simulink model "ME425HW2SIMULINK"  (R2024b)
settings: Solver=VariableStepAuto  StartTime=0.0  StopTime=simTime  RelTol=1e-3
values from neighbouring files (symbols this model uses):
  alpha_initial = pi/6    (= 0.523598775598)    [ME425HW2MATLAB.m]
  beta_initial = -pi/12    (= -0.261799387799)    [ME425HW2MATLAB.m]
  k_alpha = 3    [ME425HW2MATLAB.m]
  k_beta = -1    [ME425HW2MATLAB.m]
  k_rho = 0.45    [ME425HW2MATLAB.m]
  rho_initial = 0.5    [ME425HW2MATLAB.m]
settings Model: Creator=Arda Gencer  LastModifiedBy=Arda Gencer

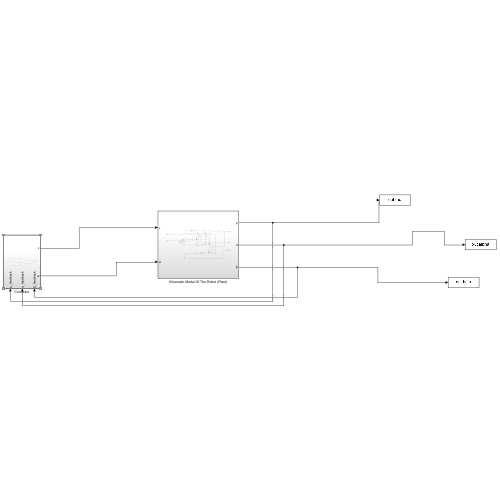
[thumbnail: Simulink's stored preview of the top-level diagram]
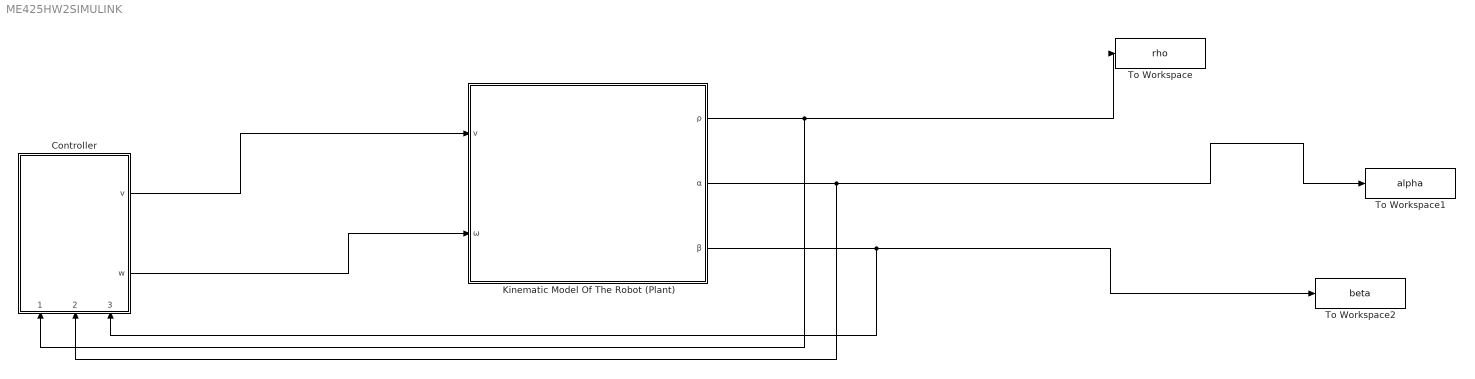
== system ME425HW2SIMULINK ==
  Controller : Subsystem
      settings: PortSchema="{\"entries\":[{\"content\":{\"sides\":[{\"content\":{},\"type\":\"ConnectorPlacement.EquallySpacedRectSide\",\"uuid\":\"75375935-2868-4b1b-a242-ab1ccb8ca21c\"},{\"content\":{\"connectorIds\":[\"Out1\",\"Out2\"],\"side\":\"RIGHT\"},\"type\":\"ConnectorPlacement.EquallySpacedRectSide\",\"uuid\":\"ed5a361e-a2c2-488a-aca6-bd0afa006ee2\"},{\"content\":{\"side\":\"TOP\"},\"type\":\"ConnectorPlacement.EquallySpacedRectSide\",\"uuid\":\"b9b83b9d-1c68-4626-97af-6a3bec3390e5\"},{\"content\":{\"connectorIds\":[\"In1\",\"In2\",\"In3\"],\"side\":\"BOTTOM\"},\"type\":\"ConnectorPlacement.EquallySpacedRectSide\",\"uuid\":\"91ac679b-6217-4ff3-855f-ef24c0e6137b\"}]},\"type\":\"ConnectorPlacement.EquallySpacedConnector\",\"uuid\":\"711fb22c-f1e8-402d-b054-03d08cfeb706\"}],\"packageUris\":[\"http://schema.mathworks.com/mf0/Connector/R2020b\"],\"version\":\"1.0\"}"
  Kinematic Model Of The Robot (Plant) : Subsystem
  To Workspace : ToWorkspace  VariableName=rho  SampleTime=-1
  To Workspace1 : ToWorkspace  VariableName=alpha  SampleTime=-1
  To Workspace2 : ToWorkspace  VariableName=beta  SampleTime=-1
  wires:
  Kinematic Model Of The Robot (Plant)/2(α) -> Controller/2(α_feedback), To Workspace1/1
  Kinematic Model Of The Robot (Plant)/1(ρ) -> Controller/1(ρ_feedback), To Workspace/1
  Kinematic Model Of The Robot (Plant)/3(β) -> Controller/3(β_feedback), To Workspace2/1
  Controller/1(v) -> Kinematic Model Of The Robot (Plant)/1(v)
  Controller/2(w) -> Kinematic Model Of The Robot (Plant)/2(ω)

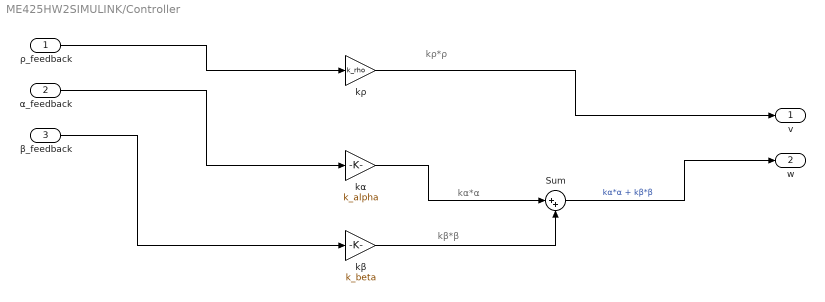
== system ME425HW2SIMULINK/Controller ==
  note: kβ*β
  note: kα*α
  note: kρ*ρ
  ρ_feedback : Inport
  α_feedback : Inport  Port=2
  β_feedback : Inport  Port=3
  Sum : Sum  Inputs=|++
  kα : Gain  Gain=k_alpha
  kβ : Gain  Gain=k_beta
  kρ : Gain  Gain=k_rho
  v : Outport
  w : Outport  Port=2
  wires:
  ρ_feedback/1 -> kρ/1
  kρ/1 -> v/1
  α_feedback/1 -> kα/1
  β_feedback/1 -> kβ/1
  kα/1 -> Sum/1
  kβ/1 -> Sum/2
  Sum/1 -> w/1  "kα*α + kβ*β"

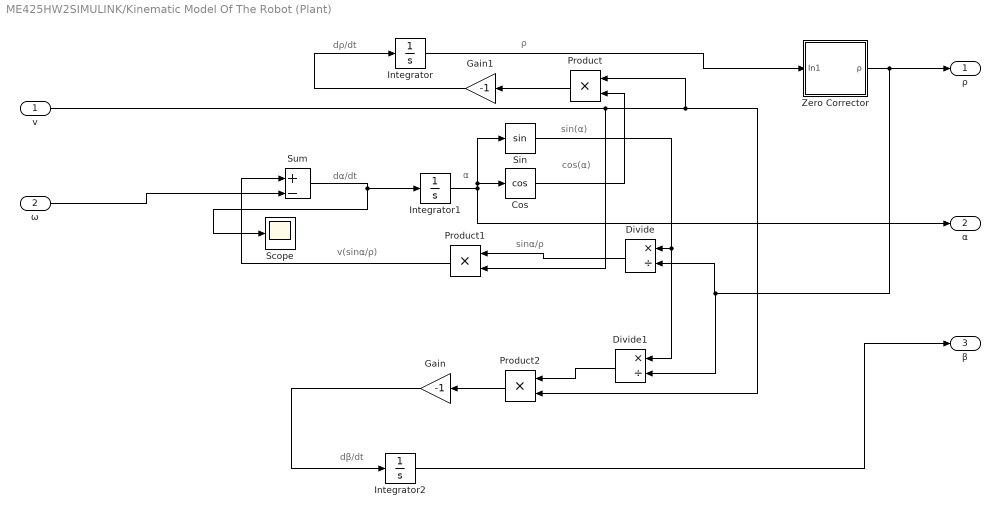
== system ME425HW2SIMULINK/Kinematic Model Of The Robot (Plant) ==
  note: dβ/dt
  note: sin(α)
  note: v(sinα/ρ)
  note: sinα/ρ
  note: ρ
  note: dα/dt
  note: dρ/dt
  note: cos(α)
  note: α
  v : Inport
  ω : Inport  Port=2
  Cos : Trigonometry  Operator=cos
  Divide : Product  Inputs=*/
  Divide1 : Product  Inputs=*/
  Gain : Gain  Gain=-1
  Gain1 : Gain  Gain=-1
  Integrator : Integrator  InitialCondition=rho_initial
  Integrator1 : Integrator  InitialCondition=alpha_initial  WrappedStateUpperValue=2*pi  WrappedStateLowerValue=0
  Integrator2 : Integrator  InitialCondition=beta_initial  WrappedStateUpperValue=2*pi  WrappedStateLowerValue=0
  Product : Product
  Product1 : Product
  Product2 : Product
  Scope : Scope
  Sin : Trigonometry
  Sum : Sum  Inputs=|+-
  Zero Corrector : Subsystem
  ρ : Outport
  α : Outport  Port=2
  β : Outport  Port=3
  wires:
  Product/1 -> Gain1/1
  Sum/1 -> Scope/1, Integrator1/1
  v/1 -> Product2/2, Product/1, Product1/2
  Cos/1 -> Product/2
  Gain/1 -> Integrator2/1
  Sin/1 -> Divide1/1, Divide/1
  Divide/1 -> Product1/1
  Integrator/1 -> Zero Corrector/1(In1)
  Integrator1/1 -> Sin/1, Cos/1, α/1
  Product2/1 -> Gain/1
  Product1/1 -> Sum/1
  Divide1/1 -> Product2/1
  Integrator2/1 -> β/1
  ω/1 -> Sum/2
  Gain1/1 -> Integrator/1
  Zero Corrector/1(ρ) -> ρ/1, Divide1/2, Divide/2

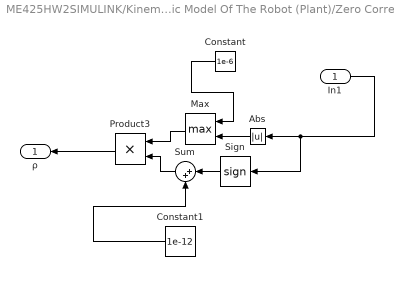
== system ME425HW2SIMULINK/Kinematic Model Of The Robot (Plant)/Zero Corrector ==
  In1 : Inport
  Abs : Abs  ZeroCross=off  SaturateOnIntegerOverflow=off
  Constant : Constant  Value=1e-6
  Constant1 : Constant  Value=1e-12
  Max : MinMax  Function=max  Inputs=2  ZeroCross=off
  Product3 : Product
  Sign : Signum  ZeroCross=off
  Sum : Sum  Inputs=|++
  ρ : Outport
  wires:
  Constant/1 -> Max/1
  Max/1 -> Product3/1
  Abs/1 -> Max/2
  In1/1 -> Sign/1, Abs/1
  Product3/1 -> ρ/1
  Sign/1 -> Sum/1
  Sum/1 -> Product3/2
  Constant1/1 -> Sum/2
